simulink model "PlantModel"  (R2021a)
settings: configuration reference "plantConfigSet" (kept outside this file)
libraries: receiver_sender x2
settings Model: DataDictionary=pathFollowingData.sldd  ParamWorkspaceSource=ReferencedWorkspace  Creator=The MathWorks, Inc.  LastModifiedBy=hgu8
settings ConfigSetRef: SourceName=plantConfigSet

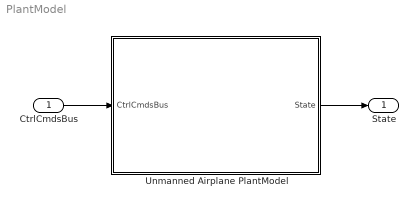
== system PlantModel ==
  CtrlCmdsBus : Inport  OutDataTypeStr=Bus: ctrlCmdsBus  SampleTime=[0.01,0]
  Unmanned Airplane PlantModel : Subsystem  TreatAsAtomicUnit=on
  State : Outport  OutDataTypeStr=Bus: FixedWingStateBus  VectorParamsAs1DForOutWhenUnconnected=off  BusOutputAsStruct=on
  wires:
  CtrlCmdsBus/1 -> Unmanned Airplane PlantModel/1(CtrlCmdsBus)
  Unmanned Airplane PlantModel/1(State) -> State/1

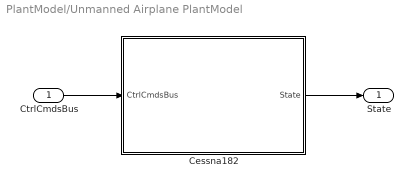
== system PlantModel/Unmanned Airplane PlantModel ==
  CtrlCmdsBus : Inport
  Cessna182 : Subsystem
  State : Outport  VectorParamsAs1DForOutWhenUnconnected=off
  wires:
  CtrlCmdsBus/1 -> Cessna182/1(CtrlCmdsBus)
  Cessna182/1(State) -> State/1

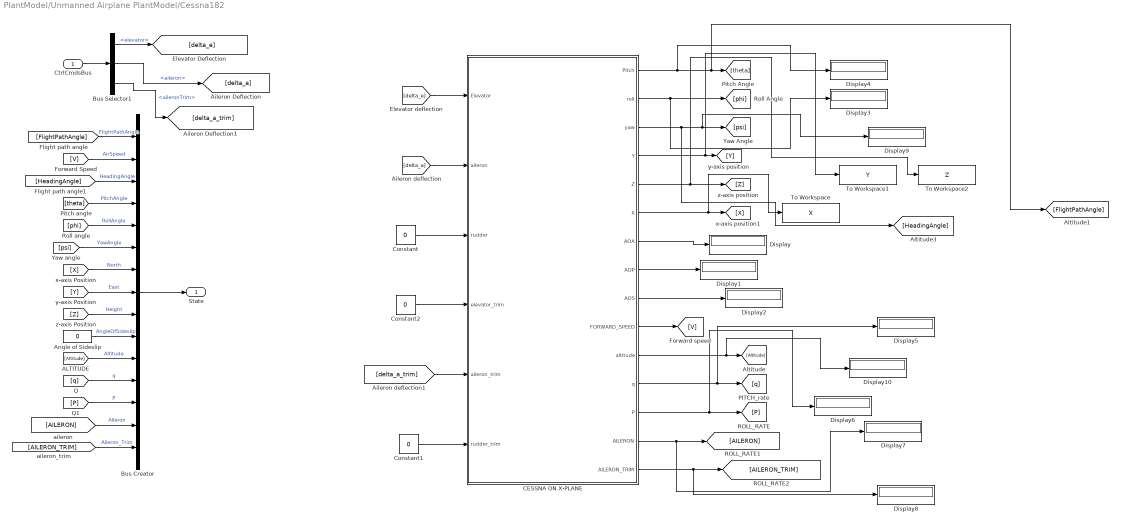
== system PlantModel/Unmanned Airplane PlantModel/Cessna182 ==
  CtrlCmdsBus : Inport  OutDataTypeStr=Bus: ctrlCmdsBus
  Angle of Sideslip : Constant  Value=0
  Bus Creator : BusCreator  Inputs=15  OutDataTypeStr=Bus: FixedWingStateBus
  Bus Selector1 : BusSelector  OutputSignals=elevator,aileron,aileronTrim
  CESSNA ON X-PLANE : Subsystem
  Constant : Constant  Value=0
  Constant1 : Constant  Value=0
  Constant2 : Constant  Value=0
  Display{,1..10} (11 alike) : Display
  To Workspace : ToWorkspace  VariableName=X  SaveFormat=Timeseries  SampleTime=-1
  To Workspace1 : ToWorkspace  VariableName=Y  SaveFormat=Timeseries  SampleTime=-1
  To Workspace2 : ToWorkspace  VariableName=Z  SaveFormat=Timeseries  SampleTime=-1
  State : Outport  OutDataTypeStr=Bus: FixedWingStateBus  VectorParamsAs1DForOutWhenUnconnected=off
  wires:
  [delta_e] -> CESSNA ON X-PLANE/1(Elevator)
  [delta_a] -> CESSNA ON X-PLANE/2(aileron)
  CESSNA ON X-PLANE/1(Pitch) -> Display4/1, [FlightPathAngle], [theta]
  CESSNA ON X-PLANE/2(roll) -> Display3/1, [phi]
  CESSNA ON X-PLANE/3(yaw) -> [HeadingAngle], Display9/1, [psi]
  CESSNA ON X-PLANE/4(Y) -> To Workspace1/1, [Y]
  CESSNA ON X-PLANE/6(X) -> To Workspace/1, [X]
  CESSNA ON X-PLANE/5(Z) -> To Workspace2/1, [Z]
  CESSNA ON X-PLANE/10(FORWARD_SPEED) -> [V]
  CESSNA ON X-PLANE/7(AOA) -> Display/1
  CESSNA ON X-PLANE/8(AOP) -> Display1/1
  CESSNA ON X-PLANE/9(AOS) -> Display2/1
  Constant/1 -> CESSNA ON X-PLANE/3(rudder)
  CESSNA ON X-PLANE/11(altitude) -> Display10/1, [Altitude]
  CESSNA ON X-PLANE/12(q) -> Display5/1, [q]
  CESSNA ON X-PLANE/13(P) -> Display6/1, [P]
  CESSNA ON X-PLANE/14(AILERON) -> Display7/1, [AILERON]
  CESSNA ON X-PLANE/15(AILERON_TRIM) -> Display8/1, [AILERON_TRIM]
  [delta_a_trim] -> CESSNA ON X-PLANE/5(aileron_trim)
  Constant2/1 -> CESSNA ON X-PLANE/4(elevator_trim)
  Constant1/1 -> CESSNA ON X-PLANE/6(rudder_trim)
  [FlightPathAngle] -> Bus Creator/1  "FlightPathAngle"
  [Z] -> Bus Creator/9  "Height"
  Angle of Sideslip/1 -> Bus Creator/10  "AngleOfSideslip"
  [X] -> Bus Creator/7  "North"
  [Y] -> Bus Creator/8  "East"
  [phi] -> Bus Creator/5  "RollAngle"
  [AILERON_TRIM] -> Bus Creator/15  "Aileron_Trim"
  [V] -> Bus Creator/2  "AirSpeed"
  [HeadingAngle] -> Bus Creator/3  "HeadingAngle"
  [P] -> Bus Creator/13  "P"
  [Altitude] -> Bus Creator/11  "Altitude"
  [psi] -> Bus Creator/6  "YawAngle"
  [AILERON] -> Bus Creator/14  "Aileron"
  [q] -> Bus Creator/12  "q"
  [theta] -> Bus Creator/4  "PitchAngle"
  Bus Creator/1 -> State/1
  CtrlCmdsBus/1 -> Bus Selector1/1
  Bus Selector1/1 -> [delta_e]  "<elevator>"
  Bus Selector1/2 -> [delta_a]  "<aileron>"
  Bus Selector1/3 -> [delta_a_trim]  "<aileronTrim>"

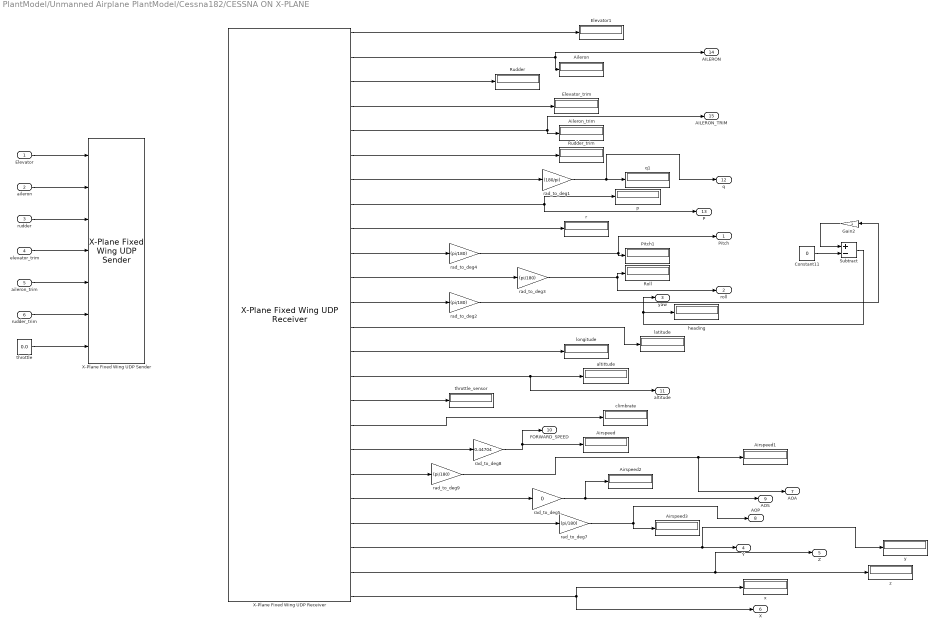
== system PlantModel/Unmanned Airplane PlantModel/Cessna182/CESSNA ON X-PLANE ==
  Elevator : Inport
  aileron : Inport  Port=2
  rudder : Inport  Port=3
  elevator_trim : Inport  Port=4
  aileron_trim : Inport  Port=5
  rudder_trim : Inport  Port=6
  Aileron : Display
  Aileron_trim : Display
  Airspeed{,1..3} (4 alike) : Display
  Constant11 : Constant  Value=0
  Elevator1 : Display
  Elevator_trim : Display
  Gain2 : Gain
  Pitch1 : Display
  Roll : Display
  Rudder : Display
  Rudder_trim : Display
  Subtract : Sum  Inputs=+-
  X-Plane Fixed Wing UDP Receiver : receiver_sender/Fixed Wing/X-Plane Fixed Wing UDP Receiver  ip_adress='127.0.0.1'  port_number=49004
  X-Plane Fixed Wing UDP Sender : receiver_sender/Fixed Wing/X-Plane Fixed Wing UDP Sender  ip_adress='127.0.0.1'  port_number=49000
  altittude : Display
  climbrate : Display
  heading : Display
  latitude : Display
  longitude : Display
  p : Display
  q1 : Display
  r : Display
  rad_to_deg1 : Gain  Gain=(180/pi)
  rad_to_deg{2..4,7,9} (5 alike) : Gain  Gain=(pi/180)
  rad_to_deg5 : Gain  Gain=0
  rad_to_deg8 : Gain  Gain=0.44704
  throttle : Constant  Value=0.0
  throttle_sensor : Display
  x : Display
  y : Display
  z : Display
  Pitch : Outport
  roll : Outport  Port=2
  yaw : Outport  Port=3
  Y : Outport  Port=4
  Z : Outport  Port=5
  X : Outport  Port=6
  AOA : Outport  Port=7
  AOP : Outport  Port=8
  AOS : Outport  Port=9
  FORWARD_SPEED : Outport  Port=10
  altitude : Outport  Port=11
  q : Outport  Port=12
  P : Outport  Port=13
  AILERON : Outport  Port=14
  AILERON_TRIM : Outport  Port=15
  wires:
  X-Plane Fixed Wing UDP Receiver/1 -> Elevator1/1
  X-Plane Fixed Wing UDP Receiver/2 -> AILERON/1, Aileron/1
  X-Plane Fixed Wing UDP Receiver/3 -> Rudder/1
  X-Plane Fixed Wing UDP Receiver/4 -> Elevator_trim/1
  X-Plane Fixed Wing UDP Receiver/5 -> AILERON_TRIM/1, Aileron_trim/1
  X-Plane Fixed Wing UDP Receiver/6 -> Rudder_trim/1
  X-Plane Fixed Wing UDP Receiver/13 -> latitude/1
  X-Plane Fixed Wing UDP Receiver/14 -> longitude/1
  X-Plane Fixed Wing UDP Receiver/15 -> altitude/1, altittude/1
  X-Plane Fixed Wing UDP Receiver/16 -> throttle_sensor/1
  X-Plane Fixed Wing UDP Receiver/17 -> climbrate/1
  Elevator/1 -> X-Plane Fixed Wing UDP Sender/1
  rudder/1 -> X-Plane Fixed Wing UDP Sender/3
  aileron/1 -> X-Plane Fixed Wing UDP Sender/2
  elevator_trim/1 -> X-Plane Fixed Wing UDP Sender/4
  rudder_trim/1 -> X-Plane Fixed Wing UDP Sender/6
  throttle/1 -> X-Plane Fixed Wing UDP Sender/7
  X-Plane Fixed Wing UDP Receiver/22 -> y/1, Y/1
  X-Plane Fixed Wing UDP Receiver/23 -> Z/1, z/1
  X-Plane Fixed Wing UDP Receiver/24 -> X/1, x/1
  rad_to_deg5/1 -> Airspeed2/1, AOS/1
  X-Plane Fixed Wing UDP Receiver/20 -> rad_to_deg5/1
  X-Plane Fixed Wing UDP Receiver/19 -> rad_to_deg9/1
  rad_to_deg9/1 -> AOA/1, Airspeed1/1
  rad_to_deg7/1 -> AOP/1, Airspeed3/1
  X-Plane Fixed Wing UDP Receiver/21 -> rad_to_deg7/1
  X-Plane Fixed Wing UDP Receiver/10 -> rad_to_deg4/1
  X-Plane Fixed Wing UDP Receiver/11 -> rad_to_deg3/1
  X-Plane Fixed Wing UDP Receiver/12 -> rad_to_deg2/1
  aileron_trim/1 -> X-Plane Fixed Wing UDP Sender/5
  X-Plane Fixed Wing UDP Receiver/18 -> rad_to_deg8/1
  rad_to_deg8/1 -> FORWARD_SPEED/1, Airspeed/1
  X-Plane Fixed Wing UDP Receiver/8 -> p/1, P/1
  X-Plane Fixed Wing UDP Receiver/9 -> r/1
  X-Plane Fixed Wing UDP Receiver/7 -> rad_to_deg1/1
  rad_to_deg1/1 -> q/1, q1/1
  rad_to_deg4/1 -> Pitch1/1, Pitch/1
  rad_to_deg3/1 -> Roll/1, roll/1
  Gain2/1 -> Subtract/1
  Constant11/1 -> Subtract/2
  rad_to_deg2/1 -> Gain2/1
  Subtract/1 -> heading/1, yaw/1
